simulink model "lab_pid"  (R2023a)
settings: Solver=VariableStepAuto  StartTime=0.0  StopTime=10.0  MaxStep=0.001  RelTol=1e-3
settings Model: Creator=Savely  LastModifiedBy=Admin

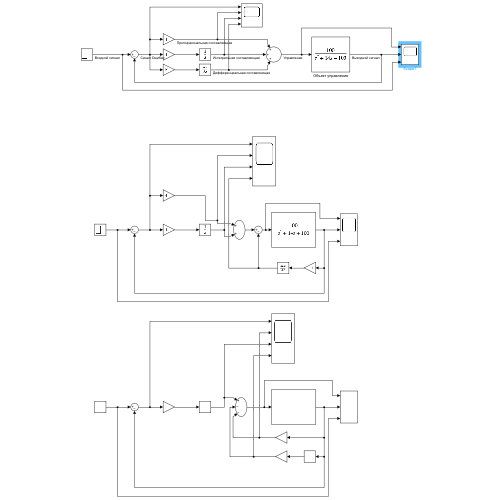
[thumbnail: Simulink's stored preview of the top-level diagram]
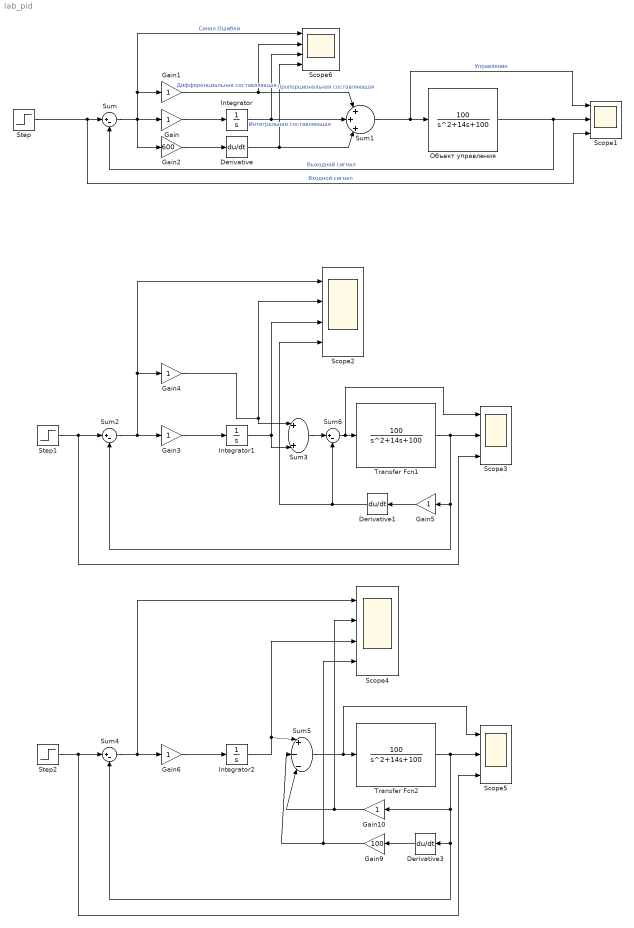
== system lab_pid ==
  Derivative : Derivative
  Derivative1 : Derivative
  Derivative3 : Derivative
  Gain{,1,3..6,10} (7 alike) : Gain
  Gain2 : Gain  Gain=600
  Gain9 : Gain  Gain=100
  Integrator : Integrator
  Integrator1 : Integrator
  Integrator2 : Integrator
  Scope1 : Scope  NumInputPorts=3
  Scope2 : Scope  NumInputPorts=4
  Scope3 : Scope  NumInputPorts=3
  Scope4 : Scope  NumInputPorts=4
  Scope5 : Scope  NumInputPorts=3
  Scope6 : Scope  NumInputPorts=4
  Step : Step  Time=0  SampleTime=0
  Step1 : Step  SampleTime=0
  Step2 : Step  SampleTime=0
  Sum{,2,4,6} (4 alike) : Sum  Inputs=|+-
  Sum1 : Sum  Inputs=|+|+|+|
  Sum3 : Sum  Inputs=|+|+|
  Sum5 : Sum  Inputs=|+|-|-|
  Transfer Fcn1 : TransferFcn  Numerator=[100]  Denominator=[1 14 100]
  Transfer Fcn2 : TransferFcn  Numerator=[100]  Denominator=[1 14 100]
  Объект управления : TransferFcn  Numerator=[100]  Denominator=[1 14 100]
  wires:
  Step/1 -> Scope1/3, Sum/1  "Входной сигнал"
  Sum/1 -> Gain2/1, Scope6/1, Gain1/1, Gain/1  "Синал Ошибки"
  Gain/1 -> Integrator/1
  Integrator/1 -> Scope6/3, Sum1/2  "Интегральная составляющая"
  Gain1/1 -> Scope6/2, Sum1/1  "Пропорциональная составляющая"
  Gain2/1 -> Derivative/1
  Derivative/1 -> Scope6/4, Sum1/3  "Дифференциальная составляющая"
  Sum1/1 -> Scope1/1, Объект управления/1  "Управление"
  Объект управления/1 -> Scope1/2, Sum/2  "Выходной сигнал"
  Sum3/1 -> Sum6/1
  Transfer Fcn1/1 -> Gain5/1, Sum2/2, Scope3/2
  Integrator1/1 -> Scope2/3, Sum3/2
  Gain3/1 -> Integrator1/1
  Gain4/1 -> Scope2/2, Sum3/1
  Derivative1/1 -> Sum6/2, Scope2/4
  Sum2/1 -> Gain4/1, Scope2/1, Gain3/1
  Step1/1 -> Scope3/3, Sum2/1
  Sum5/1 -> Scope5/1, Transfer Fcn2/1
  Transfer Fcn2/1 -> Gain10/1, Derivative3/1, Sum4/2, Scope5/2
  Integrator2/1 -> Sum5/1, Scope4/3
  Gain6/1 -> Integrator2/1
  Sum4/1 -> Scope4/1, Gain6/1
  Step2/1 -> Scope5/3, Sum4/1
  Gain5/1 -> Derivative1/1
  Sum6/1 -> Scope3/1, Transfer Fcn1/1
  Derivative3/1 -> Gain9/1
  Gain10/1 -> Sum5/3, Scope4/2
  Gain9/1 -> Scope4/4, Sum5/2
